simulink model "cic_5th_order_pipe1"  (Simulink 6.6)
settings: Solver=VariableStepDiscrete  SolverMode=SingleTasking  StartTime=0.0  StopTime=1024/100e6  RelTol=1e-3
StopFcn:
  | doFFTplot(100e6,[CIC1,CIC2,CIC3, CIC4, CIC5],['CIC1';'CIC2';'CIC3';'CIC4';'CIC5'],1,3)
  | 
  | figure
  | subplot(5,1,1)
  | plot(CIC1(1:40),'k-o','MarkerFaceColor','b');
  | legend('CIC1',1);
  | subplot(5,1,2)
  | plot(CIC2(1:40),'k-o','MarkerFaceColor','g');
  | legend('CIC2',1);
  | subplot(5,1,3)
  | plot(CIC3(1:40),'k-o','MarkerFaceColor','r');
  | legend('CIC3',1);
  | subplot(5,1,4)
  | plot(CIC4(1:40),'k-o','MarkerFaceColor','c');
  | legend('CIC4',1);
  | subplot(5,1,5)
  | plot(CIC5(1:40),'k-o','MarkerFaceColor','m');
  | legend('CIC5',1);
libraries: xbsIndex_r4 x29, simulink x4, dspsrcs4 x1
settings Model: Creator=lcrockett  LastModifiedBy=lcrockett
settings DataIOCC: SignalLoggingName=sigsOut
settings OptimizationCC: InlineParams=on  InlineInvariantSignals=on
settings DebuggingCC: SignalResolutionControl=TryResolveAllWithWarning  SolverPrmCheckMsg=none  MultiTaskDSMMsg=warning  MultiTaskCondExecSysMsg=none  StrictBusMsg=None
settings HardwareCC: TargetUnknown=on
settings RTWCC: IncludeERTFirstTime=on
settings GRTTargetCC: ModelReferenceCompliant=off  MatFileLogging=off

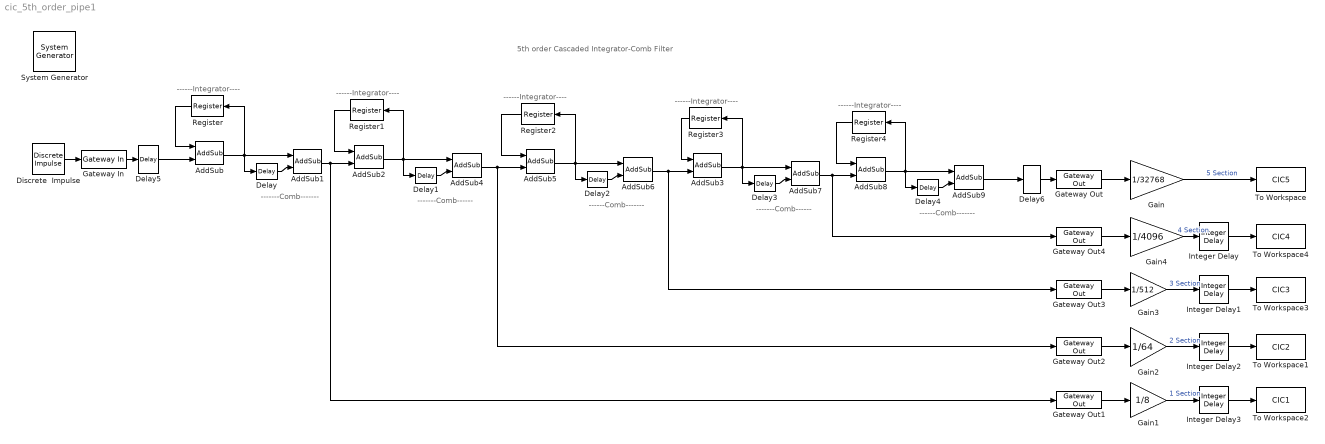
== system cic_5th_order_pipe1 ==
  note: -------Comb-------
  note: ------Integrator----
  note: ------Integrator----
  note: ------Integrator----
  note: -------Comb------
  note: ------Comb-------
  note: 5th order Cascaded Integrator-Comb Filter
  note: ------Integrator----
  note: ------Integrator----
  note: -------Comb------
  note: ------Comb-------
  " System Generator" : xbsIndex_r4/ System Generator  Tag=genX  SystemSampleTime=-1  xilinxfamily=virtex2p  part=xc2vp30  speed=-7  package=ff896  synthesis_tool=XST  clock_wrapper=Clock Enables  directory=./CIC_5th_order  testbench=off  simulink_period=1/100e6  sysclk_period=20  dcm_input_clock_period=100  incr_netlist=off  trim_vbits=Everywhere in SubSystem  dbl_ovrd=According to Block Masks  core_generation=According to Block Masks  run_coregen=off  deprecated_control=off  eval_field=0  block_type=sysgen
      settings: block_version=8.2
  AddSub : xbsIndex_r4/AddSub  mode=Addition  use_carryin=off  use_carryout=off  en=off  latency=0  precision=User Defined  arith_type="Signed  (2's comp)"  n_bits=19  bin_pt=0  quantization=Truncate  overflow=Wrap  dbl_ovrd=off  use_behavioral_HDL=on  pipelined=off  use_rpm=on  block_type=addsub
      settings: xl_area=[0, 0, 0, 0, 0, 0, 0]  block_version=VER_STRING_GOES_HERE
  AddSub1 : xbsIndex_r4/AddSub  mode=Subtraction  use_carryin=off  use_carryout=off  en=off  latency=0  precision=User Defined  arith_type="Signed  (2's comp)"  n_bits=19  bin_pt=0  quantization=Truncate  overflow=Wrap  dbl_ovrd=off  use_behavioral_HDL=on  pipelined=off  use_rpm=on  block_type=addsub
      settings: xl_area=[0, 0, 0, 0, 0, 0, 0]  block_version=VER_STRING_GOES_HERE
  AddSub2 : xbsIndex_r4/AddSub  mode=Addition  use_carryin=off  use_carryout=off  en=off  latency=0  precision=User Defined  arith_type="Signed  (2's comp)"  n_bits=22  bin_pt=0  quantization=Truncate  overflow=Wrap  dbl_ovrd=off  use_behavioral_HDL=on  pipelined=off  use_rpm=on  block_type=addsub
      settings: xl_area=[0, 0, 0, 0, 0, 0, 0]  block_version=VER_STRING_GOES_HERE
  AddSub3 : xbsIndex_r4/AddSub  mode=Addition  use_carryin=off  use_carryout=off  en=off  latency=0  precision=User Defined  arith_type="Signed  (2's comp)"  n_bits=28  bin_pt=0  quantization=Truncate  overflow=Wrap  dbl_ovrd=off  use_behavioral_HDL=on  pipelined=off  use_rpm=on  block_type=addsub
      settings: xl_area=[0, 0, 0, 0, 0, 0, 0]  block_version=VER_STRING_GOES_HERE
  AddSub4 : xbsIndex_r4/AddSub  mode=Subtraction  use_carryin=off  use_carryout=off  en=off  latency=0  precision=User Defined  arith_type="Signed  (2's comp)"  n_bits=22  bin_pt=0  quantization=Truncate  overflow=Wrap  dbl_ovrd=off  use_behavioral_HDL=on  pipelined=off  use_rpm=on  block_type=addsub
      settings: xl_area=[0, 0, 0, 0, 0, 0, 0]  block_version=VER_STRING_GOES_HERE
  AddSub5 : xbsIndex_r4/AddSub  mode=Addition  use_carryin=off  use_carryout=off  en=off  latency=0  precision=User Defined  arith_type="Signed  (2's comp)"  n_bits=25  bin_pt=0  quantization=Truncate  overflow=Wrap  dbl_ovrd=off  use_behavioral_HDL=on  pipelined=off  use_rpm=on  block_type=addsub
      settings: xl_area=[0, 0, 0, 0, 0, 0, 0]  block_version=VER_STRING_GOES_HERE
  AddSub6 : xbsIndex_r4/AddSub  mode=Subtraction  use_carryin=off  use_carryout=off  en=off  latency=0  precision=User Defined  arith_type="Signed  (2's comp)"  n_bits=25  bin_pt=0  quantization="Round  (unbiased: +/- Inf)"  overflow=Wrap  dbl_ovrd=off  use_behavioral_HDL=on  pipelined=off  use_rpm=on  block_type=addsub
      settings: xl_area=[0, 0, 0, 0, 0, 0, 0]  block_version=VER_STRING_GOES_HERE
  AddSub7 : xbsIndex_r4/AddSub  mode=Subtraction  use_carryin=off  use_carryout=off  en=off  latency=0  precision=User Defined  arith_type="Signed  (2's comp)"  n_bits=28  bin_pt=0  quantization=Truncate  overflow=Wrap  dbl_ovrd=off  use_behavioral_HDL=on  pipelined=off  use_rpm=on  block_type=addsub
      settings: xl_area=[0, 0, 0, 0, 0, 0, 0]  block_version=VER_STRING_GOES_HERE
  AddSub8 : xbsIndex_r4/AddSub  mode=Addition  use_carryin=off  use_carryout=off  en=off  latency=0  precision=User Defined  arith_type="Signed  (2's comp)"  n_bits=31  bin_pt=0  quantization=Truncate  overflow=Wrap  dbl_ovrd=off  use_behavioral_HDL=on  pipelined=off  use_rpm=on  block_type=addsub
      settings: xl_area=[0, 0, 0, 0, 0, 0, 0]  block_version=VER_STRING_GOES_HERE
  AddSub9 : xbsIndex_r4/AddSub  mode=Subtraction  use_carryin=off  use_carryout=off  en=off  latency=0  precision=User Defined  arith_type="Signed  (2's comp)"  n_bits=31  bin_pt=0  quantization="Round  (unbiased: +/- Inf)"  overflow=Wrap  dbl_ovrd=off  use_behavioral_HDL=on  pipelined=off  use_rpm=on  block_type=addsub
      settings: xl_area=[0, 0, 0, 0, 0, 0, 0]  block_version=VER_STRING_GOES_HERE
  Delay{,1..4} (5 alike) : xbsIndex_r4/Delay  en=off  latency=8  dbl_ovrd=off  reg_retiming=off  block_type=delay
      settings: infoedit=Hardware notes: A delay line is a chain, each link of which is an SRL16 followed by a flip-flop. If register retiming is enabled, the delay line is a chain of flip-flops.  xl_area=[0, 0, 0, 0, 0, 0, 0]  block_version=VER_STRING_GOES_HERE
  Delay5 : xbsIndex_r4/Delay  en=off  latency=1  dbl_ovrd=off  reg_retiming=off  block_type=delay
      settings: block_version=10.1.2
  Delay6 : xbsIndex_r4/Delay  en=off  latency=1  dbl_ovrd=off  reg_retiming=off  block_type=delay
      settings: block_version=10.1.2
  Discrete  Impulse : dspsrcs4/Discrete  Impulse  Delay=0  SampleTime=1/100e6  FrameSample=1  dataType=double  isSigned=on  wordLen=16  udDataType=sfix(16)  fracBitsMode=Best precision  numFracBits=14
  Gain : Gain  Gain=1/32768
  Gain1 : Gain  Gain=1/8
  Gain2 : Gain  Gain=1/64
  Gain3 : Gain  Gain=1/512
  Gain4 : Gain  Gain=1/4096
  Gateway In : xbsIndex_r4/Gateway In  arith_type="Signed  (2's comp)"  n_bits=16  bin_pt=0  quantization=Truncate  overflow=Flag as error  period=1/100e6  dbl_ovrd=off  timing_constraint=None  locs_specified=off  LOCs={}  block_type=gatewayin
      settings: infoedit="Gateway in block.  Converts inputs of type Simulink integer, double and fixed point to  Xilinx fixed point type.<P><P>Hardware notes:  In hardware these blocks become top level input ports."  xl_area=[0, 0, 0, 0, 0, 0, 0]  block_version=VER_STRING_GOES_HERE
  Gateway Out : xbsIndex_r4/Gateway Out  hdl_port=on  timing_constraint=None  locs_specified=off  LOCs={}  block_type=gatewayout
      settings: infoedit="Gateway out block.  Converts Xilinx fixed point inputs into ouputs of type Simulink integer, double, or fixed point.<P><P>Hardware notes:  In hardware these blocks become top level output ports or are discarded, depending on how they are configured."  xl_area=[0, 0, 0, 0, 0, 0, 0]  block_version=VER_STRING_GOES_HERE
  Gateway Out{1..4} (4 alike) : xbsIndex_r4/Gateway Out  hdl_port=off  timing_constraint=None  locs_specified=off  LOCs={}  block_type=gatewayout
      settings: infoedit="Gateway out block.  Converts Xilinx fixed point inputs into ouputs of type Simulink integer, double, or fixed point.<P><P>Hardware notes:  In hardware these blocks become top level output ports or are discarded, depending on how they are configured."  xl_area=[0, 0, 0, 0, 0, 0, 0]  block_version=VER_STRING_GOES_HERE
  Integer Delay{,1..3} (4 alike) : simulink/Discrete/Integer Delay  vinit=0.0  samptime=-1  NumDelays=1
  Register{,1..4} (5 alike) : xbsIndex_r4/Register  Orientation=left  init=0  rst=off  en=off  dbl_ovrd=off  block_type=register
      settings: xl_area=[0, 0, 0, 0, 0, 0, 0]  block_version=VER_STRING_GOES_HERE
  To Workspace : ToWorkspace  VariableName=CIC5  SampleTime=-1  SaveFormat=Array
  To Workspace1 : ToWorkspace  VariableName=CIC2  SampleTime=-1  SaveFormat=Array
  To Workspace2 : ToWorkspace  VariableName=CIC1  SampleTime=-1  SaveFormat=Array
  To Workspace3 : ToWorkspace  VariableName=CIC3  SampleTime=-1  SaveFormat=Array
  To Workspace4 : ToWorkspace  VariableName=CIC4  SampleTime=-1  SaveFormat=Array
  wires:
  Register/1 -> AddSub/1
  AddSub/1 -> Register/1, Delay/1, AddSub1/1
  Delay/1 -> AddSub1/2
  Register1/1 -> AddSub2/1
  AddSub2/1 -> Register1/1, Delay1/1, AddSub4/1
  Delay1/1 -> AddSub4/2
  AddSub1/1 -> AddSub2/2, Gateway Out1/1
  Register2/1 -> AddSub5/1
  AddSub5/1 -> Register2/1, Delay2/1, AddSub6/1
  Delay2/1 -> AddSub6/2
  AddSub4/1 -> AddSub5/2, Gateway Out2/1
  Gateway In/1 -> Delay5/1
  Discrete  Impulse/1 -> Gateway In/1
  Gateway Out1/1 -> Gain1/1
  Gateway Out2/1 -> Gain2/1
  Gateway Out/1 -> Gain/1
  Gain/1 -> To Workspace/1  "5 Section"
  Gain1/1 -> Integer Delay3/1  "1 Section"
  Gain2/1 -> Integer Delay2/1  "2 Section"
  Register3/1 -> AddSub3/1
  AddSub3/1 -> Register3/1, Delay3/1, AddSub7/1
  Delay3/1 -> AddSub7/2
  AddSub6/1 -> AddSub3/2, Gateway Out3/1
  Register4/1 -> AddSub8/1
  AddSub8/1 -> Register4/1, Delay4/1, AddSub9/1
  Delay4/1 -> AddSub9/2
  AddSub7/1 -> AddSub8/2, Gateway Out4/1
  AddSub9/1 -> Delay6/1
  Gateway Out3/1 -> Gain3/1
  Gateway Out4/1 -> Gain4/1
  Gain3/1 -> Integer Delay1/1  "3 Section"
  Gain4/1 -> Integer Delay/1  "4 Section"
  Delay5/1 -> AddSub/2
  Delay6/1 -> Gateway Out/1
  Integer Delay/1 -> To Workspace4/1
  Integer Delay1/1 -> To Workspace3/1
  Integer Delay2/1 -> To Workspace1/1
  Integer Delay3/1 -> To Workspace2/1
